simulink model "simexa29"  (Simulink 3.00)
settings: Solver=ode23  SolverMode=SingleTasking  StartTime=0.0  StopTime=20  MaxStep=0.1  RelTol=1e-3  AbsTol=1e-3
settings Model: SaveTime=off  SaveOutput=off  RTWTemplateMakefile=grt_vc.tmf

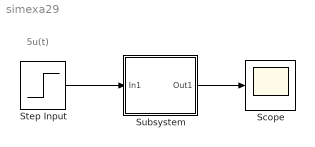
== system simexa29 ==
  note: 5u(t)
  Scope : Scope
      settings: TickLabels=on  TimeRange=auto  YMin=-5  YMax=5  SaveToWorkspace=off  SaveName=ScopeData  DataFormat=Matrix
  Step Input : Step  Time=0  Before=0  After=5  SampleTime=0
  Subsystem : Subsystem
  wires:
  Subsystem/1(Out1) -> Scope/1
  Step Input/1 -> Subsystem/1(In1)

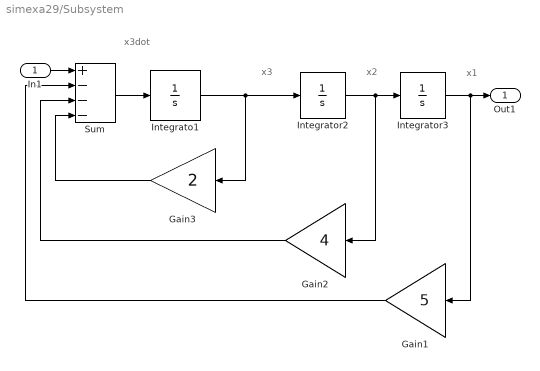
== system simexa29/Subsystem ==
  note: x3dot
  note: x1
  note: x2
  note: x3
  In1 : Inport  Port=1  PortWidth=-1  SampleTime=-1  DataType=auto
      settings: SignalType=auto
  Gain1 : Gain  Orientation=left  Gain=5  SaturateOnIntegerOverflow=on
  Gain2 : Gain  Orientation=left  Gain=4  SaturateOnIntegerOverflow=on
  Gain3 : Gain  Orientation=left  Gain=2  SaturateOnIntegerOverflow=on
  Integrato1 : Integrator  ExternalReset=none  InitialConditionSource=internal  InitialCondition=0  LimitOutput=off  UpperSaturationLimit=inf  LowerSaturationLimit=-inf  ShowSaturationPort=off  ShowStatePort=off  AbsoluteTolerance=auto
  Integrator2 : Integrator  ExternalReset=none  InitialConditionSource=internal  InitialCondition=0  LimitOutput=off  UpperSaturationLimit=inf  LowerSaturationLimit=-inf  ShowSaturationPort=off  ShowStatePort=off  AbsoluteTolerance=auto
  Integrator3 : Integrator  ExternalReset=none  InitialConditionSource=internal  InitialCondition=0  LimitOutput=off  UpperSaturationLimit=inf  LowerSaturationLimit=-inf  ShowSaturationPort=off  ShowStatePort=off  AbsoluteTolerance=auto
  Sum : Sum  Inputs=+---  SaturateOnIntegerOverflow=on
  Out1 : Outport  Port=1
  wires:
  Integrator3/1 -> Gain1/1, Out1/1
  Integrator2/1 -> Gain2/1, Integrator3/1
  Gain1/1 -> Sum/2
  Gain2/1 -> Sum/3
  Gain3/1 -> Sum/4
  Integrato1/1 -> Gain3/1, Integrator2/1
  Sum/1 -> Integrato1/1
  In1/1 -> Sum/1
